simulink model "SIGNAL"  (R2020a)
settings: Solver=VariableStepAuto  StartTime=0.0  StopTime=5000  RelTol=1e-3
settings Model: Creator=86150  LastModifiedBy=86150

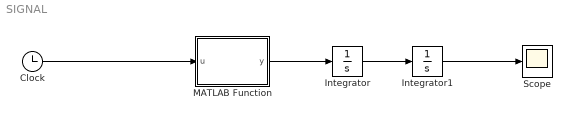
== system SIGNAL ==
  Clock : Clock
  Integrator : Integrator
  Integrator1 : Integrator
  MATLAB Function : MATLAB Function  TreatAsAtomicUnit=on
  Scope : Scope
  wires:
  Clock/1 -> MATLAB Function/1(u)
  MATLAB Function/1(y) -> Integrator/1
  Integrator/1 -> Integrator1/1
  Integrator1/1 -> Scope/1

== matlab function SIGNAL/MATLAB Function ==
  data: u input; y output
function y = fcn(u)

y = 0.5*u+sin(u);
